simulink model "DC_DC_BoostConverter"  (Simulink 7.0)
settings: Solver=ode23t  StartTime=0.0  StopTime=0.08  MaxStep=1.e-06  MinStep=1.e-08  RelTol=1e-3
libraries: powerlib x9, simulink x1
settings Model: Creator=sc  LastModifiedBy=sc
settings SolverCC: InitialStep=1.e-07

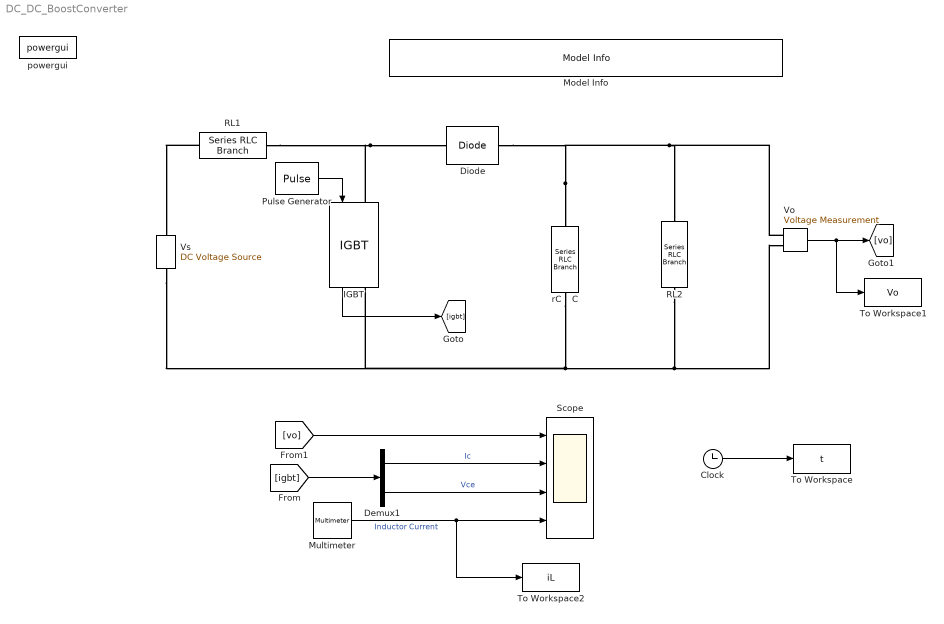
== system DC_DC_BoostConverter ==
  " RL1" : powerlib/Elements/Series RLC Branch  DialogController=POWERSYS.PowerSysDialog  PhysicalDomain=powersysdomain  SubClassName=unknown  LeftPortType=p1  RightPortType=p1  LConnTagsString=__new0  RConnTagsString=__new0  BranchType=RL  Resistance=0.1  Inductance=1.e-3  SetiL0=off  InitialCurrent=0  Capacitance=1.0  Setx0=off  InitialVoltage=0  Measurements=Branch current
  " RL2" : powerlib/Elements/Series RLC Branch  Orientation=down  DialogController=POWERSYS.PowerSysDialog  PhysicalDomain=powersysdomain  SubClassName=unknown  LeftPortType=p1  RightPortType=p1  LConnTagsString=__new0  RConnTagsString=__new0  BranchType=R  Resistance=100  Inductance=1e-3  SetiL0=off  InitialCurrent=0  Capacitance=1.e-04  Setx0=off  InitialVoltage=0  Measurements=Branch current
  " rC    C" : powerlib/Elements/Series RLC Branch  Orientation=down  DialogController=POWERSYS.PowerSysDialog  PhysicalDomain=powersysdomain  SubClassName=unknown  LeftPortType=p1  RightPortType=p1  LConnTagsString=__new0  RConnTagsString=__new0  BranchType=RC  Resistance=0.01  Inductance=1e-3  SetiL0=off  InitialCurrent=0  Capacitance=50.e-05  Setx0=off  InitialVoltage=0  Measurements=Branch current
  Clock : Clock
      settings: Decimation=10
  Demux1 : Demux  Outputs=2
  Diode : powerlib/Power Electronics/Diode  DialogController=POWERSYS.PowerSysDialog  SystemSampleTime=-1  Ron=0.01  Lon=0  Vf=0.8  IC=0  Rs=500  Cs=250e-9  Measurements=off
  IGBT : powerlib/Power Electronics/IGBT  Orientation=down  DialogController=POWERSYS.PowerSysDialog  SystemSampleTime=-1  Ron=0.001  Lon=0  Vf=1  Tf=1e-6  Tt=2e-6  IC=0  Rs=500  Cs=1.e-7  Measurements=on
  Model Info : simulink/Model-Wide Utilities/Model Info  SystemSampleTime=-1  InitialBlockCM=None  BlockCM=None  Frame=on  DisplayStringWithTags=DC-DC Boost Converter (DC-DC Step-up converter)  HorizontalTextAlignment=Center  LeftAlignmentValue=0.5  SourceBlockDiagram=DC_DC_BoostConverter  TagMaxNumber=20
  Multimeter : powerlib/Measurements/Multimeter  SystemSampleTime=-1  PhasorSimulation=off  OutputType=Complex  sel=1  L=3  Gain=1  yselected="{'Ib:  RL1'};"  PSBOutputType=1  PSBequivalent=0  AxesSetting=[0,0.1,-100,100]  Display=0  SavedBlockNames=-11
  Pulse Generator : DiscretePulseGenerator  PulseType=Time based  Period=10.e-05  PulseWidth=60
  Scope : Scope  NumInputPorts=4
      settings: TimeRange=0.02  YMin=-50~-50~-50~0  YMax=150~100~150~60  SaveName=var  MaxDataPoints=100000
  To Workspace : ToWorkspace  VariableName=t  SampleTime=-1  SaveFormat=Array
  To Workspace1 : ToWorkspace  VariableName=Vo  SampleTime=-1  SaveFormat=Array
  To Workspace2 : ToWorkspace  VariableName=iL  SampleTime=-1  SaveFormat=Array
  Vo : powerlib/Measurements/Voltage Measurement  DialogController=POWERSYS.PowerSysDialog  SystemSampleTime=-1  PhasorSimulation=off  OutputType=Complex  PSBequivalent=0
  Vs : powerlib/Electrical Sources/DC Voltage Source  Orientation=up  DialogController=POWERSYS.PowerSysDialog  SystemSampleTime=-1  Amplitude=12  Measurements=None
  powergui : powerlib/powergui  SystemSampleTime=-1  SimulationMode=Continuous  SampleTime=50e-6  echomessages=off  RestoreLinks=warning  x0status=blocks  Frange=[0:2:500]  Ylog=off  Xlog=on  ShowGrid=off  save=off  variable=ZData  ZoomFFT=on  StartTime=0.0  cycles=1  DisplayStyle=1  fundamental=60  FreqAxis=off  MaxFrequency=1000  frequencyindice=0  frequencyindicesteady=1  RmsSteady=1  display=off  Ts=0  frequency=60  methode=off  HookPort=off  Interpol=off  SPID=off  FunctionMessages=off
  wires:
  IGBT/1 -> [igbt]
  [igbt] -> Demux1/1
  Vo/1 -> [vo], To Workspace1/1
  [vo] -> Scope/1
  Demux1/1 -> Scope/2  "Ic"
  Demux1/2 -> Scope/3  "Vce"
  Multimeter/1 -> Scope/4, To Workspace2/1  "Inductor Current"
  Pulse Generator/1 -> IGBT/1
  Clock/1 -> To Workspace/1
  connections:
  Vs/LConn1 -- IGBT/RConn1 -- " rC    C"/RConn1 -- Vo/LConn2 -- " RL2"/RConn1
  Vo/LConn1 -- " rC    C"/LConn1 -- Diode/RConn1 -- " RL2"/LConn1
  IGBT/LConn1 -- Diode/LConn1 -- " RL1"/RConn1
  " RL1"/LConn1 -- Vs/RConn1
